simulink model "ex_blocchi_elementi_discontinui"  (R2024b)
settings: Solver=VariableStepAuto  StartTime=0.0  StopTime=10  RelTol=1e-3

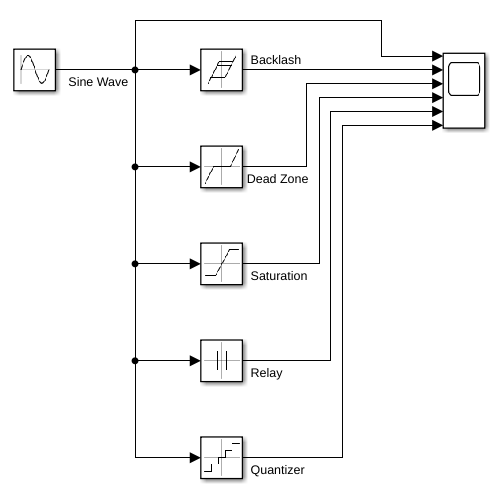
[thumbnail: Simulink's stored preview of the top-level diagram]
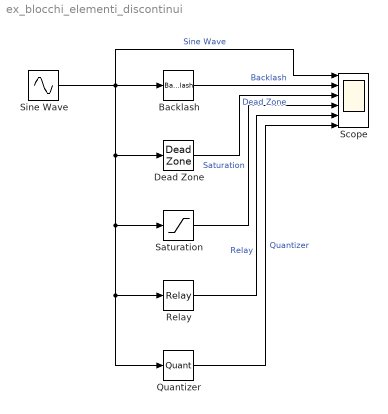
== system ex_blocchi_elementi_discontinui ==
  Backlash : Backlash
  Dead Zone : DeadZone
  Quantizer : Quantizer  QuantizationInterval=0.1
  Relay : Relay
  Saturation : Saturate
  Scope : Scope  NumInputPorts=6
  Sine Wave : Sin  SampleTime=0
  wires:
  Sine Wave/1 -> Quantizer/1, Relay/1, Saturation/1, Dead Zone/1, Scope/1, Backlash/1  "Sine Wave"
  Backlash/1 -> Scope/2  "Backlash"
  Dead Zone/1 -> Scope/3  "Dead Zone"
  Saturation/1 -> Scope/4  "Saturation"
  Relay/1 -> Scope/5  "Relay"
  Quantizer/1 -> Scope/6  "Quantizer"
